simulink model "Robot_diferencial_cinematica"  (R2017b)
settings: Solver=VariableStepAuto  StartTime=0.0  StopTime=Tsim  MaxStep=1e-2  MinStep=1e-5  RelTol=1e-3
values from neighbouring files (symbols this model uses):
  Amp = 2    [graf.m]
  CI = [0 0 atan(A)]    [graf.m]
  frec = 5    [graf.m]
settings Model: Creator=Raúl  LastModifiedBy=Alvaro

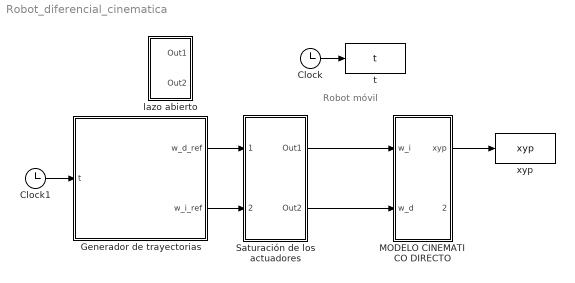
== system Robot_diferencial_cinematica ==
  note: Robot móvil
  Clock : Clock
  Clock1 : Clock
  Generador de trayectorias : Subsystem
  MODELO CINEMATICO DIRECTO : Subsystem
  Saturación de los actuadores : Subsystem
  lazo abierto : Subsystem
  t : ToWorkspace  VariableName=t  SampleTime=-1
  xyp : ToWorkspace  VariableName=xyp  SampleTime=-1
  wires:
  MODELO CINEMATICO DIRECTO/1(xyp) -> xyp/1
  Clock/1 -> t/1
  Clock1/1 -> Generador de trayectorias/1(t)
  Saturación de los actuadores/2(Out2) -> MODELO CINEMATICO DIRECTO/2(w_d)
  Saturación de los actuadores/1(Out1) -> MODELO CINEMATICO DIRECTO/1(w_i)
  Generador de trayectorias/1(w_d_ref) -> Saturación de los actuadores/1(w_i_ref)
  Generador de trayectorias/2(w_i_ref) -> Saturación de los actuadores/2(w_d_ref)

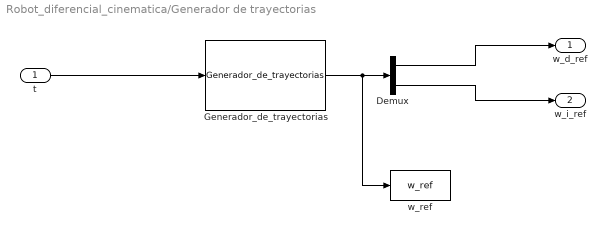
== system Robot_diferencial_cinematica/Generador de trayectorias ==
  t : Inport
  Demux : Demux  Outputs=2
  Generador_de_trayectorias : MATLABFcn  MATLABFcn=Generador_de_trayectorias
  w_ref : ToWorkspace  VariableName=w_ref  SampleTime=-1
  w_d_ref : Outport
  w_i_ref : Outport  Port=2
  wires:
  Generador_de_trayectorias/1 -> w_ref/1, Demux/1
  t/1 -> Generador_de_trayectorias/1
  Demux/2 -> w_i_ref/1
  Demux/1 -> w_d_ref/1

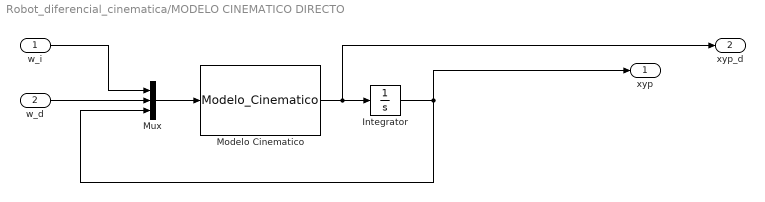
== system Robot_diferencial_cinematica/MODELO CINEMATICO DIRECTO ==
  w_i : Inport
  w_d : Inport  Port=2
  Integrator : Integrator  InitialCondition=CI
  "Modelo Cinematico " : MATLABFcn  MATLABFcn=Modelo_Cinematico
  Mux : Mux  Inputs=3
  xyp : Outport
  xyp_d : Outport  Port=2
  wires:
  "Modelo Cinematico "/1 -> xyp_d/1, Integrator/1
  w_i/1 -> Mux/1
  Integrator/1 -> xyp/1, Mux/3
  Mux/1 -> "Modelo Cinematico "/1
  w_d/1 -> Mux/2

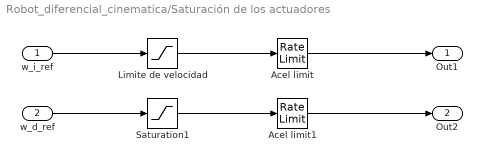
== system Robot_diferencial_cinematica/Saturación de los actuadores ==
  w_i_ref : Inport
  w_d_ref : Inport  Port=2
  Acel limit : RateLimiter  RisingSlewLimit=2.5  FallingSlewLimit=-2.5  SampleTimeMode=inherited
  Acel limit1 : RateLimiter  RisingSlewLimit=2.5  FallingSlewLimit=-2.5  SampleTimeMode=inherited
  Limite de velocidad : Saturate  UpperLimit=2.5  LowerLimit=-2.5
  Saturation1 : Saturate  UpperLimit=2.5  LowerLimit=-2.5
  Out1 : Outport
  Out2 : Outport  Port=2
  wires:
  w_i_ref/1 -> Limite de velocidad/1
  w_d_ref/1 -> Saturation1/1
  Limite de velocidad/1 -> Acel limit/1
  Acel limit/1 -> Out1/1
  Saturation1/1 -> Acel limit1/1
  Acel limit1/1 -> Out2/1

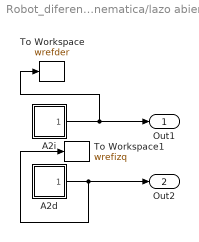
== system Robot_diferencial_cinematica/lazo abierto ==
  A2d : Subsystem
  A2i : Subsystem
  To Workspace : ToWorkspace  VariableName=wrefder  SampleTime=-1
  To Workspace1 : ToWorkspace  VariableName=wrefizq  SampleTime=-1
  Out1 : Outport
  Out2 : Outport  Port=2
  wires:
  A2i/1(Out1) -> Out1/1, To Workspace/1
  A2d/1(Out1) -> Out2/1, To Workspace1/1

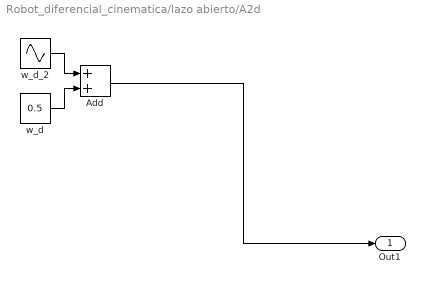
== system Robot_diferencial_cinematica/lazo abierto/A2d ==
  Add : Sum
  w_d : Constant  Value=0.5
  w_d_2 : Sin  Amplitude=Amp  Frequency=frec  Phase=pi  SampleTime=0
  Out1 : Outport
  wires:
  Add/1 -> Out1/1
  w_d_2/1 -> Add/1
  w_d/1 -> Add/2

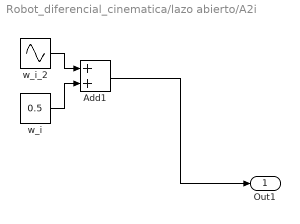
== system Robot_diferencial_cinematica/lazo abierto/A2i ==
  Add1 : Sum
  w_i : Constant  Value=0.5
  w_i_2 : Sin  Amplitude=Amp  Frequency=frec  SampleTime=0
  Out1 : Outport
  wires:
  w_i/1 -> Add1/2
  w_i_2/1 -> Add1/1
  Add1/1 -> Out1/1
